simulink model "MIAC_ZTransform_PLC_Coder"  (R2018b)
settings: Solver=FixedStepDiscrete  StartTime=0.0  StopTime=5.5*10^4  FixedStep=1  RelTol=1e-3
libraries: peGeneralControl x2, simulink x1, slident x1
settings Model: Creator=Trips  LastModifiedBy=Trips
settings ConfigComp: PLC_TargetIDE=step7  PLC_GenerateReport=off  PLC_LaunchReport=off

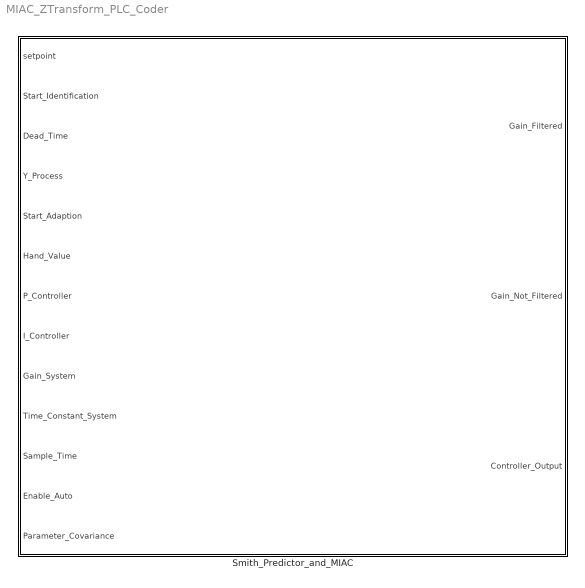
== system MIAC_ZTransform_PLC_Coder ==
  Smith_Predictor_and_MIAC : Subsystem  TreatAsAtomicUnit=on  SystemSampleTime=1

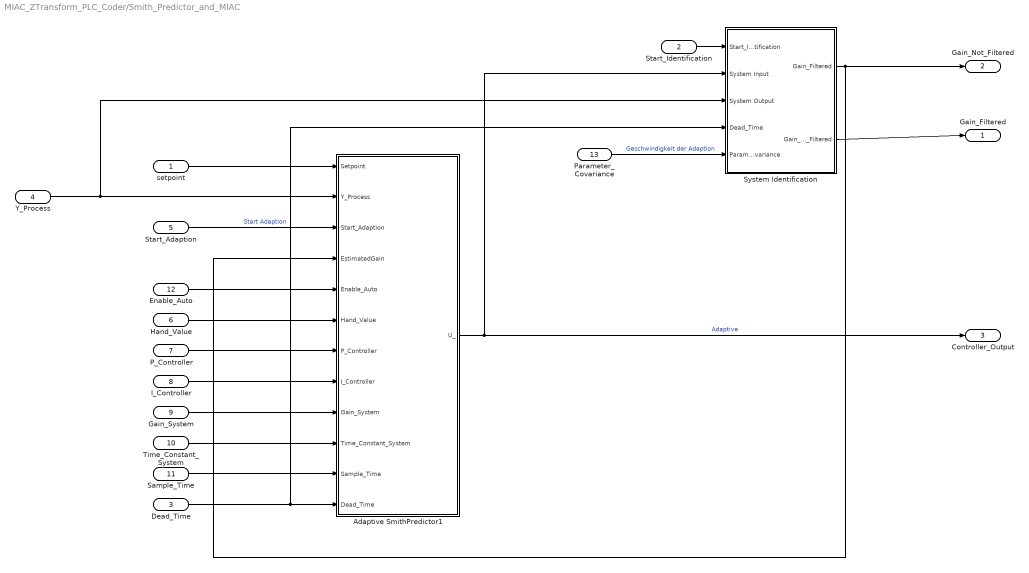
== system MIAC_ZTransform_PLC_Coder/Smith_Predictor_and_MIAC ==
  setpoint : Inport
  Start_Identification : Inport  Port=2
  Dead_Time : Inport  Port=3
  Y_Process : Inport  Port=4
  Start_Adaption : Inport  Port=5
  Hand_Value : Inport  Port=6
  P_Controller : Inport  Port=7
  I_Controller : Inport  Port=8
  Gain_System : Inport  Port=9
  Time_Constant_System : Inport  Port=10
  Sample_Time : Inport  Port=11
  " Enable_Auto" : Inport  Port=12
  Parameter_Covariance : Inport  Port=13
  Adaptive SmithPredictor1 : Subsystem
  System Identification : Subsystem  TreatAsAtomicUnit=on  SystemSampleTime=1
  Gain_Filtered : Outport
  Gain_Not_Filtered : Outport  Port=2
  Controller_Output : Outport  Port=3
  wires:
  Gain_System/1 -> Adaptive SmithPredictor1/9(Gain_System)
  Dead_Time/1 -> Adaptive SmithPredictor1/12(" Dead_Time"), System Identification/4(Dead_Time)
  Adaptive SmithPredictor1/1(U_) -> System Identification/2(System Input), Controller_Output/1  "Adaptive"
  Time_Constant_System/1 -> Adaptive SmithPredictor1/10(Time_Constant_System)
  P_Controller/1 -> Adaptive SmithPredictor1/7(P_Controller)
  Sample_Time/1 -> Adaptive SmithPredictor1/11(Sample_Time)
  Parameter_Covariance/1 -> System Identification/5(Parameter_Covariance)  "Geschwindigkeit der Adaption"
  I_Controller/1 -> Adaptive SmithPredictor1/8(I_Controller)
  Start_Adaption/1 -> Adaptive SmithPredictor1/3(Start_Adaption)  "Start Adaption"
  System Identification/2(Gain_Not_Filtered) -> Gain_Filtered/1
  setpoint/1 -> Adaptive SmithPredictor1/1(Setpoint)
  Start_Identification/1 -> System Identification/1(Start_Identification)
  System Identification/1(Gain_Filtered) -> Adaptive SmithPredictor1/4(EstimatedGain), Gain_Not_Filtered/1
  " Enable_Auto"/1 -> Adaptive SmithPredictor1/5(Enable_Auto)
  Hand_Value/1 -> Adaptive SmithPredictor1/6(Hand_Value)
  Y_Process/1 -> System Identification/3(System Output), Adaptive SmithPredictor1/2(Y_Process)

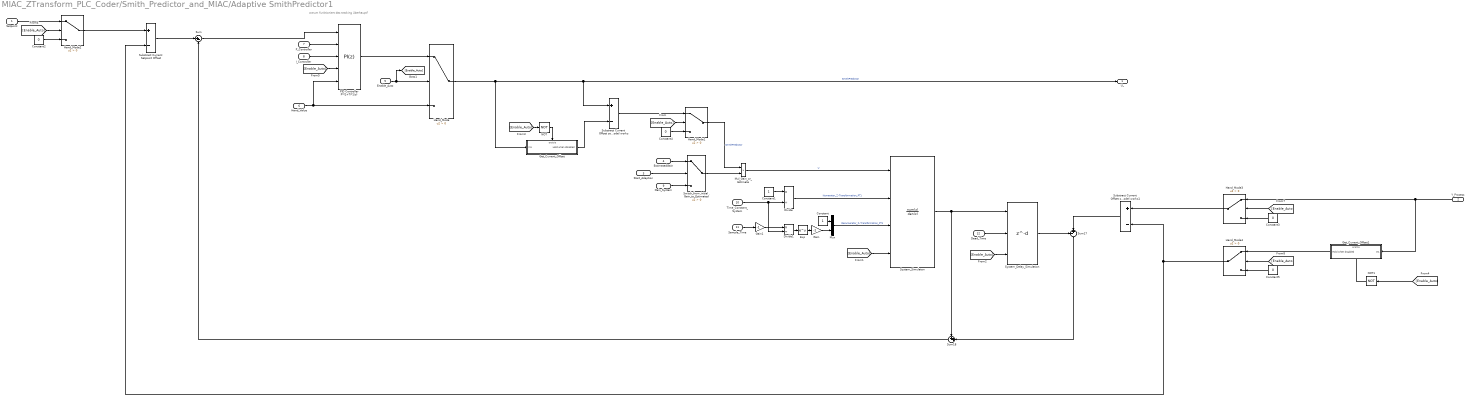
== system MIAC_ZTransform_PLC_Coder/Smith_Predictor_and_MIAC/Adaptive SmithPredictor1 ==
  note: warum funktioniert das tracking überhaupt?
  Setpoint : Inport
  Y_Process : Inport  Port=2
  Start_Adaption : Inport  Port=3
  EstimatedGain : Inport  Port=4
  Enable_Auto : Inport  Port=5
  Hand_Value : Inport  Port=6
  P_Controller : Inport  Port=7
  I_Controller : Inport  Port=8
  Gain_System : Inport  Port=9
  Time_Constant_System : Inport  Port=10
  Sample_Time : Inport  Port=11
  " Dead_Time" : Inport  Port=12
  Constant : Constant
  Constant1 : Constant
  Constant{2..5} (4 alike) : Constant  Value=0
  Divide : Product  Inputs=*/
  Divide1 : Product  Inputs=*/
  Exp : Math  SaturateOnIntegerOverflow=on
  Gain : Gain  Gain=-1
  Gain1 : Gain  Gain=-1
  Get_Current_Offset : Subsystem
  Get_Current_Offset1 : Subsystem
  Hand_Mode{,1..4} (5 alike) : Switch  Criteria=u2 > Threshold
  Mul_Gain_or_Estimate : Product
  Mux : Mux  Inputs=2
  NOT : Logic  Operator=NOT  IconShape=distinctive  AllPortsSameDT=off  OutDataTypeStr=boolean
  NOT1 : Logic  Operator=NOT  IconShape=distinctive  AllPortsSameDT=off  OutDataTypeStr=boolean
  PID Controller P*(1+Ti*1/s) : simulink/Continuous/PID Controller  Controller=PI  Form=Parallel  TimeDomain=Discrete-time  SampleTime=1  IntegratorMethod=Forward Euler  FilterMethod=Forward Euler  ControllerParametersSource=external  P=3.04732259067536  I=0.00445689106465138  D=118.272348286844  UseFilter=on  N=0.00420306193364532  TunerSelectOption=Transfer Function Based (PID Tuner App)  InitialConditionSource=external  InitialConditionForIntegrator=0  InitialConditionForFilter=0  DifferentiatorICPrevScaledInput=0  ExternalReset=rising  TrackingMode=off  Kt=1  LimitOutput=on  UpperSaturationLimit=100  LowerSaturationLimit=0  LinearizeAsGain=on  AntiWindupMode=none  Kb=1  POutMin=[]  POutMax=[]  IOutMin=[]  IOutMax=[]  DOutMin=[]  DOutMax=[]  NOutMin=[]  NOutMax=[]  SumOutMin=[]  SumOutMax=[]  SaturationOutMin=[]  SaturationOutMax=[]  PParamMin=[]  PParamMax=[]  IParamMin=[]  IParamMax=[]  DParamMin=[]  DParamMax=[]  NParamMin=[]  NParamMax=[]  KbParamMin=[]  KbParamMax=[]  KtParamMin=[]  KtParamMax=[]  KbOutMin=[]  KbOutMax=[]  KtOutMin=[]  KtOutMax=[]  IntegratorOutMin=[]  IntegratorOutMax=[]  FilterOutMin=[]  FilterOutMax=[]  SumI1OutMin=[]  SumI1OutMax=[]  SumI2OutMin=[]  SumI2OutMax=[]  SumI3OutMin=[]  SumI3OutMax=[]  SumI4OutMin=[]  SumI4OutMax=[]  SumDOutMin=[]  SumDOutMax=[]  DifferentiatorOutMin=[]  DifferentiatorOutMax=[]  FilterDiffOutCoefMin=[]  FilterDiffOutCoefMax=[]  ReciprocalOutMin=[]  ReciprocalOutMax=[]  SumDenOutMin=[]  SumDenOutMax=[]  SumNumOutMin=[]  SumNumOutMax=[]  DivideOutMin=[]  DivideOutMax=[]  IntegratorContinuousStateAttributes=''  IntegratorStateMustResolveToSignalObject=off  IntegratorRTWStateStorageClass=Auto  FilterContinuousStateAttributes=''  FilterStateMustResolveToSignalObject=off  FilterRTWStateStorageClass=Auto  ParallelPVariant=ExternalParameters  IdealPVariant=Disabled  IVariant=ExternalParameters  DVariant=Disabled  IntegratorVariant=Discrete  SatVariant=Enabled  AWVariant=Passthrough  PCopyVariant=Disabled  TRVariant=Disabled  FdbkBlocksVariant=Forward  IdealPFdbkVariant=Disabled  SatFdbkVariant=Disabled  DerivativeFilterVariant=Disabled  NVariant=Disabled  NCopyVariant=Disabled_SignalSpec  FilterICVariant=Disabled  IntegratorICVariant=ExternalICs  ExternalResetVariant=ExternalReset  TRSumVariant=Passthrough  SumFdbkVariant=Disabled  SumVariant=Sum_PI
  Substract Current Offset so that the linearised model works : Sum  Inputs=+-
  Substract Current Offset so that the linearised model works1 : Sum  Inputs=+-
  Substract Current Setpoint Offset : Sum  Inputs=+-
  Sum : Sum  Inputs=|+-
  Sum17 : Sum  Inputs=-+|
  Sum18 : Sum  Inputs=++|
  Switch_from_initial_Gain_to_Estimated : Switch  Criteria=u2 > Threshold
  System_Delay_Simulation : Delay  DelayLengthSource=Input port  DelayLength=600  DelayLengthUpperLimit=800  ExternalReset=Rising  SampleTime=1
      settings: InputPortMap=u0,p1,r5
  System_Simulaton : DiscreteTransferFcn  NumeratorSource=Input port  DenominatorSource=Input port  ExternalReset=Rising  SampleTime=1  a0EqualsOne=on
      settings: InputPortMap=u0,p1,p3,r7
  U_ : Outport
  wires:
  Substract Current Setpoint Offset/1 -> Sum/1
  Sum/1 -> PID Controller P*(1+Ti*1/s)/1
  Hand_Mode/1 -> U_/1, Substract Current Offset so that the linearised model works/1, Get_Current_Offset/1(In1)  "SmithPredictor"
  Substract Current Offset so that the linearised model works1/1 -> Sum17/2
  System_Simulaton/1 -> Sum18/1, System_Delay_Simulation/1
  System_Delay_Simulation/1 -> Sum17/1
  Sum17/1 -> Sum18/2
  Mul_Gain_or_Estimate/1 -> System_Simulaton/1  "U"
  Switch_from_initial_Gain_to_Estimated/1 -> Mul_Gain_or_Estimate/2
  PID Controller P*(1+Ti*1/s)/1 -> Hand_Mode/1
  Hand_Value/1 -> PID Controller P*(1+Ti*1/s)/5, Hand_Mode/3
  Enable_Auto/1 -> [Enable_Auto], Hand_Mode/2
  P_Controller/1 -> PID Controller P*(1+Ti*1/s)/2
  I_Controller/1 -> PID Controller P*(1+Ti*1/s)/3
  Divide/1 -> System_Simulaton/2  "Numerator_Z-Transformation_PT1"
  Mux/1 -> System_Simulaton/3  "Denumerator_Z-Transformation_PT1"
  Time_Constant_System/1 -> Divide1/2, Divide/2
  Constant/1 -> Mux/1
  Exp/1 -> Gain/1
  Gain/1 -> Mux/2
  Divide1/1 -> Exp/1
  Sample_Time/1 -> Gain1/1
  " Dead_Time"/1 -> System_Delay_Simulation/2
  Gain_System/1 -> Switch_from_initial_Gain_to_Estimated/3
  Start_Adaption/1 -> Switch_from_initial_Gain_to_Estimated/2
  EstimatedGain/1 -> Switch_from_initial_Gain_to_Estimated/1
  Constant1/1 -> Divide/1
  Gain1/1 -> Divide1/1
  [Enable_Auto] -> Hand_Mode1/2
  Hand_Mode1/1 -> Mul_Gain_or_Estimate/1  "SmithPredictor"
  Constant4/1 -> Hand_Mode1/3
  [Enable_Auto] -> System_Simulaton/4
  [Enable_Auto] -> System_Delay_Simulation/3
  Substract Current Offset so that the linearised model works/1 -> Hand_Mode1/1
  Get_Current_Offset/1(Hold when disabled) -> Substract Current Offset so that the linearised model works/2
  [Enable_Auto] -> NOT/1
  NOT/1 -> Get_Current_Offset/Enable
  Sum18/1 -> Sum/2
  Hand_Mode2/1 -> Substract Current Setpoint Offset/1
  NOT1/1 -> Get_Current_Offset1/Enable
  [Enable_Auto] -> NOT1/1
  Hand_Mode4/1 -> Substract Current Setpoint Offset/2, Substract Current Offset so that the linearised model works1/2
  [Enable_Auto] -> PID Controller P*(1+Ti*1/s)/4
  Setpoint/1 -> Hand_Mode2/1
  [Enable_Auto] -> Hand_Mode2/2
  Constant2/1 -> Hand_Mode2/3
  Y_Process/1 -> Get_Current_Offset1/1(In1), Hand_Mode3/1
  [Enable_Auto] -> Hand_Mode3/2
  Constant3/1 -> Hand_Mode3/3
  Hand_Mode3/1 -> Substract Current Offset so that the linearised model works1/1
  Constant5/1 -> Hand_Mode4/3
  [Enable_Auto] -> Hand_Mode4/2
  Get_Current_Offset1/1(Hold when disabled) -> Hand_Mode4/1

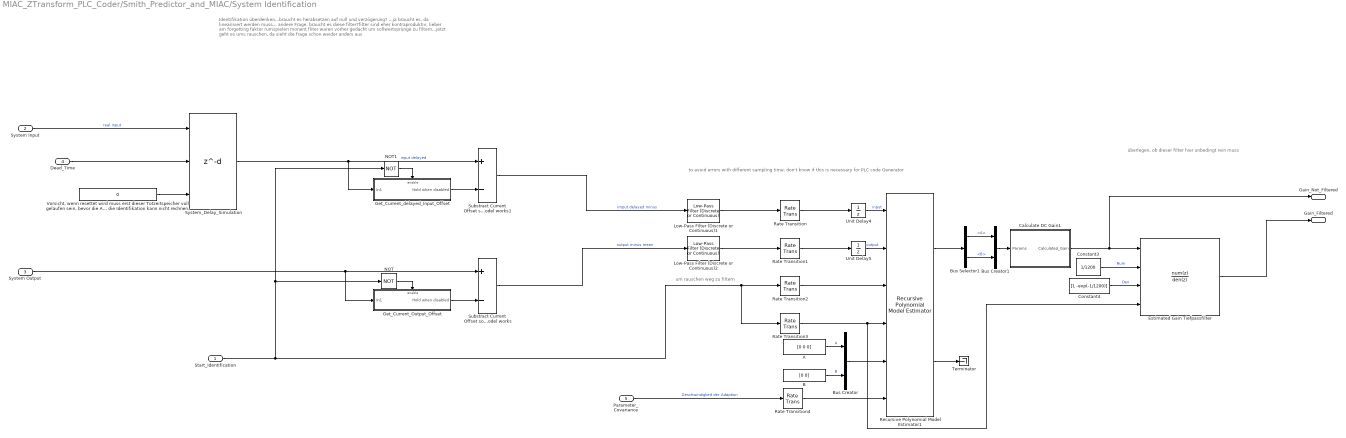
== system MIAC_ZTransform_PLC_Coder/Smith_Predictor_and_MIAC/System Identification ==
  note: um rauschen weg zu filtern
  note: überlegen, ob dieser filter hier unbedingt rein muss
  note: Identifikation überdenken...braucht es herabsetzen auf null und verzögerung?
      | ...ja braucht es, da linearisiert werden muss...
      |
      | andere Frage, braucht es diese filter?filter sind eher kontraproduktiv, lieber am forgetting faktor rumspielen
      | monent fliter waren vorher gedacht um sollwertsprünge zu filtern...jetzt geht es ums rauschen, da sieht die frage schon weider anders aus
  note: to avoid errors with different sampling time, don't know if this is necessary for PLC code Generator
  Start_Identification : Inport
  System Input : Inport  Port=2
  System Output : Inport  Port=3
  Dead_Time : Inport  Port=4
  Parameter_Covariance : Inport  Port=5
  A : Constant  Value=[0 0 0]  VectorParams1D=off
  B : Constant  Value=[0 0]  VectorParams1D=off
  Bus Creator : BusCreator  Inputs=2
  Bus Creator1 : BusCreator  Inputs=2
  Bus Selector1 : BusSelector  OutputSignals=A,B
  Calculate DC Gain1 : Subsystem
  Constant3 : Constant  Value=1/1200
  Constant4 : Constant  Value=[1 -exp(-1/1200)]
  Estimated Gain Tiefpassfilter : DiscreteTransferFcn  NumeratorSource=Input port  DenominatorSource=Input port  ExternalReset=Rising  a0EqualsOne=on
      settings: InputPortMap=u0,p1,p3,r7
  Get_Current_Output_Offset : Subsystem
  Get_Current_delayed_Input_Offset : Subsystem
  Low-Pass Filter (Discrete or Continuous)1 : peGeneralControl/Low-Pass Filter (Discrete or Continuous)  K=1  T=100  B=inf  A=-inf  Ts=-1
  Low-Pass Filter (Discrete or Continuous)2 : peGeneralControl/Low-Pass Filter (Discrete or Continuous)  K=1  T=100  B=inf  A=-inf  Ts=-1
  NOT : Logic  Operator=NOT  IconShape=distinctive  AllPortsSameDT=off  OutDataTypeStr=boolean
  NOT1 : Logic  Operator=NOT  IconShape=distinctive  AllPortsSameDT=off  OutDataTypeStr=boolean
  Rate Transition{,1..4} (5 alike) : RateTransition  OutPortSampleTime=1
  Recursive Polynomial Model Estimator1 : slident/Estimators/Recursive Polynomial Model Estimator  ModelStructure=ARX  InitialEstimateSource=External  A0=2  B0=1  C0=1  D0=1  F0=1  nk=1  P0=100  InitialInputs=0  InitialOutputs=0  History=Infinite  WindowLength=2000  EstimationMethod=Forgetting Factor  AdaptationParameter=1  HasTimeVaryingAdaptationParameter=off  NormalizationBias=eps  OutputError=on  OutputP=off  AddEnablePort=on  ExternalReset=Rising  InputProcessing=Sample-based  Ts=1
      settings: SourceProductName=System Identification Toolbox  SourceProductBaseCode=ID
  Substract Current Offset so that the linearised model works : Sum  Inputs=+-
  Substract Current Offset so that the linearised model works1 : Sum  Inputs=+-
  System_Delay_Simulation : Delay  DelayLengthSource=Input port  DelayLength=600  DelayLengthUpperLimit=800  ExternalReset=Rising  SampleTime=1
      settings: InputPortMap=u0,p1,r5
  Terminator : Terminator
  Unit Delay4 : UnitDelay  InitialCondition=[0]
  Unit Delay5 : UnitDelay
  "Vorsicht, wenn resettet wird muss erst dieser Totzeitspeicher voll gelaufen sein, bevor die Adaption starten darf! Sonst kommt heir immer 0 raus und die Identifikation kann nicht rechnen." : Constant  Value=0
  Gain_Filtered : Outport
  Gain_Not_Filtered : Outport  Port=2
  wires:
  Recursive Polynomial Model Estimator1/1 -> Bus Selector1/1
  Unit Delay4/1 -> Recursive Polynomial Model Estimator1/1  "input"
  Unit Delay5/1 -> Recursive Polynomial Model Estimator1/2  "output"
  Rate Transition/1 -> Unit Delay4/1
  Rate Transition1/1 -> Unit Delay5/1
  Bus Creator1/1 -> Calculate DC Gain1/1(Params)
  Bus Selector1/1 -> Bus Creator1/1  "<A>"
  Bus Selector1/2 -> Bus Creator1/2  "<B>"
  Rate Transition2/1 -> Recursive Polynomial Model Estimator1/3
  Rate Transition3/1 -> Recursive Polynomial Model Estimator1/4, Estimated Gain Tiefpassfilter/4
  Substract Current Offset so that the linearised model works/1 -> Low-Pass Filter (Discrete or Continuous)2/1  "output minus mean"
  NOT/1 -> Get_Current_Output_Offset/Enable
  Get_Current_Output_Offset/1(Hold when disabled) -> Substract Current Offset so that the linearised model works/2
  System Output/1 -> Get_Current_Output_Offset/1(In1), Substract Current Offset so that the linearised model works/1
  Get_Current_delayed_Input_Offset/1(Hold when disabled) -> Substract Current Offset so that the linearised model works1/2
  NOT1/1 -> Get_Current_delayed_Input_Offset/Enable
  Recursive Polynomial Model Estimator1/2 -> Terminator/1
  Start_Identification/1 -> NOT/1, NOT1/1, Rate Transition3/1, Rate Transition2/1
  Estimated Gain Tiefpassfilter/1 -> Gain_Filtered/1
  Low-Pass Filter (Discrete or Continuous)1/1 -> Rate Transition/1
  Low-Pass Filter (Discrete or Continuous)2/1 -> Rate Transition1/1
  System Input/1 -> System_Delay_Simulation/1  "real input"
  "Vorsicht, wenn resettet wird muss erst dieser Totzeitspeicher voll gelaufen sein, bevor die Adaption starten darf! Sonst kommt heir immer 0 raus und die Identifikation kann nicht rechnen."/1 -> System_Delay_Simulation/3
  Dead_Time/1 -> System_Delay_Simulation/2
  Substract Current Offset so that the linearised model works1/1 -> Low-Pass Filter (Discrete or Continuous)1/1  "imput delayed minus"
  System_Delay_Simulation/1 -> Substract Current Offset so that the linearised model works1/1, Get_Current_delayed_Input_Offset/1(In1)  "input delayed"
  Calculate DC Gain1/1(Calculated_Gain) -> Gain_Not_Filtered/1, Estimated Gain Tiefpassfilter/1
  Constant3/1 -> Estimated Gain Tiefpassfilter/2  "Num"
  Constant4/1 -> Estimated Gain Tiefpassfilter/3  "Den"
  Parameter_Covariance/1 -> Rate Transition4/1  "Geschwindigkeit der Adaption"
  Bus Creator/1 -> Recursive Polynomial Model Estimator1/5
  A/1 -> Bus Creator/1  "A"
  B/1 -> Bus Creator/2  "B"
  Rate Transition4/1 -> Recursive Polynomial Model Estimator1/6

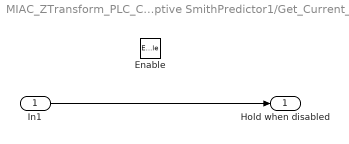
== system MIAC_ZTransform_PLC_Coder/Smith_Predictor_and_MIAC/Adaptive SmithPredictor1/Get_Current_Offset ==
  In1 : Inport
  Enable : EnablePort
  Hold when disabled : Outport
  wires:
  In1/1 -> Hold when disabled/1

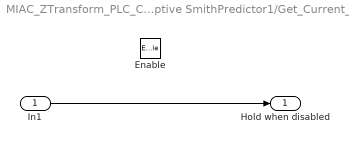
== system MIAC_ZTransform_PLC_Coder/Smith_Predictor_and_MIAC/Adaptive SmithPredictor1/Get_Current_Offset1 ==
  In1 : Inport
  Enable : EnablePort
  Hold when disabled : Outport
  wires:
  In1/1 -> Hold when disabled/1

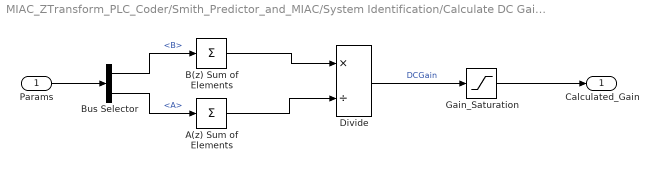
== system MIAC_ZTransform_PLC_Coder/Smith_Predictor_and_MIAC/System Identification/Calculate DC Gain1 ==
  Params : Inport
  A(z) Sum of Elements : Sum  Inputs=+
  B(z) Sum of Elements : Sum  Inputs=+
  Bus Selector : BusSelector  OutputSignals=B,A
  Divide : Product  Inputs=*/
  Gain_Saturation : Saturate  UpperLimit=1.5  LowerLimit=0.01
  Calculated_Gain : Outport
  wires:
  Params/1 -> Bus Selector/1
  Bus Selector/1 -> B(z) Sum of Elements/1  "<B>"
  Bus Selector/2 -> A(z) Sum of Elements/1  "<A>"
  B(z) Sum of Elements/1 -> Divide/1
  Divide/1 -> Gain_Saturation/1  "DCGain"
  A(z) Sum of Elements/1 -> Divide/2
  Gain_Saturation/1 -> Calculated_Gain/1

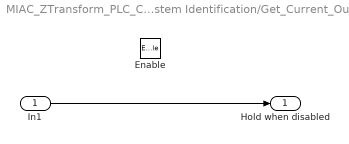
== system MIAC_ZTransform_PLC_Coder/Smith_Predictor_and_MIAC/System Identification/Get_Current_Output_Offset ==
  In1 : Inport
  Enable : EnablePort
  Hold when disabled : Outport
  wires:
  In1/1 -> Hold when disabled/1

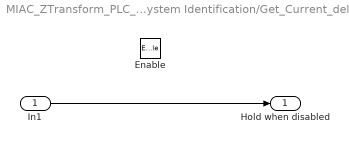
== system MIAC_ZTransform_PLC_Coder/Smith_Predictor_and_MIAC/System Identification/Get_Current_delayed_Input_Offset ==
  In1 : Inport
  Enable : EnablePort
  Hold when disabled : Outport
  wires:
  In1/1 -> Hold when disabled/1
